simulink model "simple_walk_2d_robot"  (R2014b)
settings: Solver=FixedStepDiscrete  StartTime=0.0  StopTime=inf  FixedStep=sample_time  RelTol=1e-3
InitFcn:
  | tg.sampletime = correctedSampleTime;
settings Model: SimulationMode=external  BufferReuse=off  Creator=wmartin  LastModifiedBy=drl
settings SolverCC: EnableConcurrentExecution=on
settings DataIOCC: LimitDataPoints=off  MaxDataPoints=1e7  SaveFormat=StructureWithTime  SignalLogging=off  DSMLogging=off
settings OptimizationCC: BlockReduction=off  OptimizeBlockIOStorage=off  BufferReuse=off  GlobalBufferReuse=off  ExpressionFolding=off  ExpressionDepthLimit=2147483647  LocalBlockOutputs=off  SimCompilerOptimization=On
settings DebuggingCC: UnderspecifiedInitializationDetection=Classic  MergeDetectMultiDrivingBlocksExec=none  StateNameClashWarn=warning
settings HardwareCC: ProdIntDivRoundTo=Zero  ProdEndianess=LittleEndian  ProdLongLongMode=on  ProdHWDeviceType=Generic->32-bit x86 compatible
settings ModelReferenceCC: UpdateModelReferenceTargets=IfOutOfDate  ModelReferenceNumInstancesAllowed=Single  ModelReferenceMinAlgLoopOccurrences=on
settings RTWCC: SystemTargetFile=slrt.tlc  TemplateMakefile=slrt_default_tmf  Description=Simulink Real-Time  RTWVerbose=off  ProcessScript=slrt_make_rtw_hook  RTWCompilerOptimization=On
settings CodeAppCC: MaxIdLength=256
settings SimulinkRealTimeCC: GeneratePreprocessorConditionals=Disable all  EnableShiftOperators=on  RL32LogBufSizeModifier=1e8

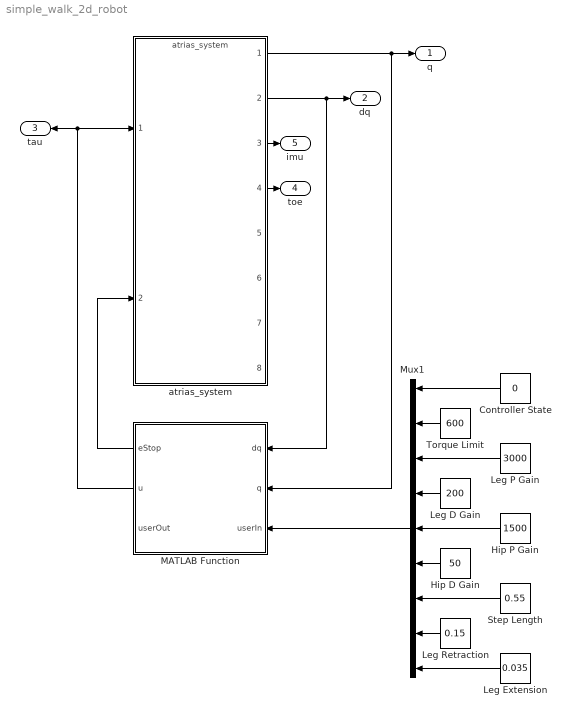
== system simple_walk_2d_robot ==
  Controller State : Constant  Value=0
  Hip D Gain : Constant  Value=50
  Hip P Gain : Constant  Value=1500
  Leg D Gain : Constant  Value=200
  Leg Extension : Constant  Value=0.035
  Leg P Gain : Constant  Value=3000
  Leg Retraction : Constant  Value=0.15
  MATLAB Function : MATLAB Function  TreatAsAtomicUnit=on
  Mux1 : Mux  Inputs=9
  Step Length : Constant  Value=0.55
  Torque Limit : Constant  Value=600
  atrias_system : ModelReference  ModelNameDialog=atrias_system  SimulationMode=Normal  ModelReferenceVersion=1.2418  CopyOfModelName=atrias_system  DefaultDataLogging=on
  q : Outport
  dq : Outport  Port=2
  tau : Outport  Port=3
  toe : Outport  Port=4
  imu : Outport  Port=5
  wires:
  atrias_system/2 -> dq/1, MATLAB Function/1(dq)
  atrias_system/1 -> q/1, MATLAB Function/2(q)
  MATLAB Function/1(eStop) -> atrias_system/2
  MATLAB Function/2(u) -> tau/1, atrias_system/1
  atrias_system/4 -> toe/1
  Mux1/1 -> MATLAB Function/3(userIn)
  Controller State/1 -> Mux1/1
  Torque Limit/1 -> Mux1/2
  Leg P Gain/1 -> Mux1/3
  Leg D Gain/1 -> Mux1/4
  Hip P Gain/1 -> Mux1/5
  Hip D Gain/1 -> Mux1/6
  atrias_system/3 -> imu/1
  Step Length/1 -> Mux1/7
  Leg Extension/1 -> Mux1/9
  Leg Retraction/1 -> Mux1/8

== matlab function simple_walk_2d_robot/MATLAB Function ==
  data: dq input; eStop output; q input; u output; userIn input; userOut output
function [eStop, u, userOut] = wrapper(dq, q, userIn)
%WRAPPER Controller wrapper.
%
% Notes:
% 	- State indexes (rBl rBm rAl rAm lBl lBm lAl lAm rHm lHm bR bY bP) 
%   - Input indexes (rB rA rH lB lA lH)

    % Actual controller function
    [eStop, u, userOut] = controller(q, dq, userIn);
end % wrapper
